simulink model "kalman_filter_design"  (R2023b)
settings: Solver=VariableStepAuto  StartTime=0.0  StopTime=20  MaxStep=0.01  RelTol=1e-3
undefined symbols (not defined in the file): Discrete, Rotation_Local, t_sample, t_sample_camera, Time, Wheel_Speed_to_Motor_Speed
libraries: simulink_extras x5, simulink x4, sharedTrackingLibrary x1, ctrlSharedLib x1
settings Model: Creator=ander  LastModifiedBy=ander

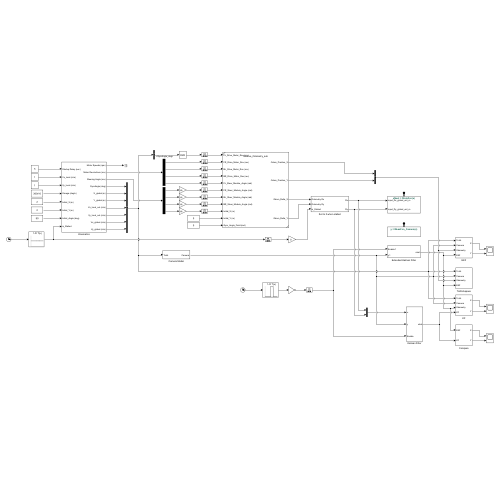
[thumbnail: Simulink's stored preview of the top-level diagram]
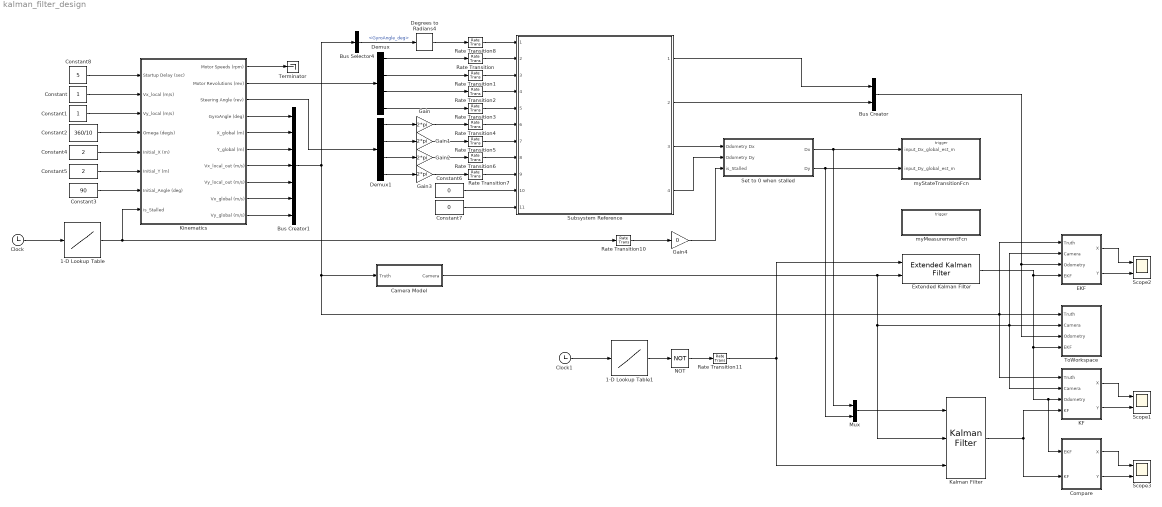
== system kalman_filter_design ==
  1-D Lookup Table : Lookup_n-D  NumberOfTableDimensions=1  BreakpointsForDimension1=[0 7 7.1 10 10.1 15]  Table=[0 0 1 1 0 0]*0  InternalRulePriority=Speed  RndMeth=Simplest
  1-D Lookup Table1 : Lookup_n-D  NumberOfTableDimensions=1  BreakpointsForDimension1=[0 7 7.1 10 10.1 15]  Table=[0 0 1 1 0 0]  InternalRulePriority=Speed  RndMeth=Simplest
  Bus Creator : BusCreator  Inputs=2
  Bus Creator1 : BusCreator  Inputs=7
  Bus Selector4 : BusSelector  OutputSignals=GyroAngle_deg
  Camera Model : Subsystem
  Clock : Clock
  Clock1 : Clock
  Compare : Subsystem
  Constant : Constant
  Constant1 : Constant
  Constant2 : Constant  Value=360/10
  Constant3 : Constant  Value=90
  Constant4 : Constant  Value=2
  Constant5 : Constant  Value=2
  Constant6 : Constant  Value=0
  Constant7 : Constant  Value=0
  Constant8 : Constant  Value=5
  Degrees to Radians4 : simulink_extras/Transformations/Degrees to Radians
  Demux : Demux
  Demux1 : Demux
  EKF : Subsystem
  Extended Kalman Filter : sharedTrackingLibrary/Extended Kalman Filter  StateTransitionFcn=StateFcn  HasStateTransitionJacobianFcn=off  HasAdditiveProcessNoise=Additive  ProcessNoise=1e-3*eye(2)  HasTimeVaryingProcessNoise=off  HasStateTransitionFcnExtraArgument=0  InitialState=[0;0]  InitialStateCovariance=1e-3*eye(2)  MeasurementFcn1=MeasFcn_Camera  HasMeasurementJacobianFcn1=off  HasMeasurementEnablePort1=on  HasAdditiveMeasurementNoise1=Additive  MeasurementNoise1=0.1*eye(2)  HasTimeVaryingMeasurementNoise1=off  HasMeasurementFcnExtraArgument1=0  HasMeasurementWrapping1=off  MeasurementFcn2=MeasFcn_IMU  HasMeasurementJacobianFcn2=off  HasMeasurementEnablePort2=off  HasAdditiveMeasurementNoise2=Additive  MeasurementNoise2=1e-4*eye(2)  HasTimeVaryingMeasurementNoise2=off  HasMeasurementFcnExtraArgument2=0  HasMeasurementWrapping2=off  MeasurementFcn3=myMeasurementFcn  HasMeasurementJacobianFcn3=off  HasMeasurementEnablePort3=off  HasAdditiveMeasurementNoise3=Additive  MeasurementNoise3=1  HasTimeVaryingMeasurementNoise3=off  HasMeasurementFcnExtraArgument3=0  HasMeasurementWrapping3=off  MeasurementFcn4=myMeasurementFcn  HasMeasurementJacobianFcn4=off  HasMeasurementEnablePort4=off  HasAdditiveMeasurementNoise4=Additive  MeasurementNoise4=1  HasTimeVaryingMeasurementNoise4=off  HasMeasurementFcnExtraArgument4=0  HasMeasurementWrapping4=off  MeasurementFcn5=myMeasurementFcn  HasMeasurementJacobianFcn5=off  HasMeasurementEnablePort5=off  HasAdditiveMeasurementNoise5=Additive  MeasurementNoise5=1  HasTimeVaryingMeasurementNoise5=off  HasMeasurementFcnExtraArgument5=0  HasMeasurementWrapping5=off  EnableMultirate=off  StateTransitionFcnSampleTime=t_sample  MeasurementFcn1SampleTime=t_sample_camera  MeasurementFcn2SampleTime=t_sample  MeasurementFcn3SampleTime=1  MeasurementFcn4SampleTime=1  MeasurementFcn5SampleTime=1  UseCurrentEstimator=on  OutputStateCovariance=off  DataType=double  SampleTime=t_sample  NumberOfMeasurements=1
  Gain{,1..3} (4 alike) : Gain  Gain=2*pi
  Gain4 : Gain  Gain=0
  KF : Subsystem
  Kalman Filter : ctrlSharedLib/Kalman Filter  TimeDomain=Discrete-Time  UseCurrentEstimator=on  ModelSource=Individual A, B, C, D matrices  ModelSourceVariable=ss(0.95,1,1,0,1)  A=eye(2)  B=eye(2)  C=eye(2)  D=eye(2)*0  NumberOfStates=1  NumberOfInputs=1  NumberOfOutputs=1  InitialEstimateSource=Dialog  X0=[0;0]  P0=10  UseK=off  UseGH=off  NumberOfProcessNoiseInputs=1  G=eye(2)  TimeInvariantG=on  H=eye(2)*1e-2  TimeInvariantH=on  Q=1e-3*eye(2)  TimeInvariantQ=on  R=0.1*eye(2)  TimeInvariantR=on  N=0  TimeInvariantN=on  AddInputPort=on  AddEnablePort=on  OutputEstimatedY=off  OutputP=off  Ts=-1
  Kinematics : Subsystem
  Mux : Mux  Inputs=2
  NOT : Logic  Operator=NOT  IconShape=distinctive  AllPortsSameDT=off  OutDataTypeStr=boolean
  Rate Transition{,1..8,10..11} (11 alike) : RateTransition  OutPortSampleTime=t_sample
  Scope1 : Scope  NumInputPorts=2
  Scope2 : Scope  NumInputPorts=2
  Scope3 : Scope  NumInputPorts=2
  Set to 0 when stalled : Subsystem
  Subsystem Reference : Subsystem  ReferencedSubsystem=Swerve_Odometry_sub
  Terminator : Terminator
  ToWorkspace : Subsystem
  myMeasurementFcn : Subsystem  TreatAsAtomicUnit=on
  myStateTransitionFcn : Subsystem  TreatAsAtomicUnit=on
  wires:
  Kinematics/2(Motor Revolutions (rev)) -> Demux/1
  Kinematics/1(Motor Speeds (rpm)) -> Terminator/1
  Kinematics/3(Steering Angle (rev)) -> Demux1/1
  Demux/3 -> Rate Transition2/1
  Demux/2 -> Rate Transition1/1
  Demux/4 -> Rate Transition3/1
  Demux/1 -> Rate Transition/1
  Constant3/1 -> Kinematics/7(Initial_Angle (deg))
  Rate Transition/1 -> Subsystem Reference/2
  Rate Transition1/1 -> Subsystem Reference/3
  Rate Transition2/1 -> Subsystem Reference/4
  Rate Transition3/1 -> Subsystem Reference/5
  Rate Transition4/1 -> Subsystem Reference/6
  Rate Transition5/1 -> Subsystem Reference/7
  Rate Transition6/1 -> Subsystem Reference/8
  Rate Transition7/1 -> Subsystem Reference/9
  Rate Transition8/1 -> Subsystem Reference/1
  Constant4/1 -> Kinematics/5(Initial_X (m))
  Constant5/1 -> Kinematics/6(Initial_Y (m))
  Subsystem Reference/1 -> Bus Creator/1
  Bus Creator1/1 -> Bus Selector4/1, KF/1(Truth), EKF/1(Truth), ToWorkspace/1(Truth), Camera Model/1(Truth)
  Bus Creator/1 -> EKF/3(Odometry), ToWorkspace/3(Odometry)
  Demux1/3 -> Gain2/1
  Demux1/2 -> Gain1/1
  Demux1/1 -> Gain/1
  Degrees to Radians4/1 -> Rate Transition8/1
  Gain/1 -> Rate Transition4/1
  Demux1/4 -> Gain3/1
  Gain1/1 -> Rate Transition5/1
  Gain2/1 -> Rate Transition6/1
  Gain3/1 -> Rate Transition7/1
  Extended Kalman Filter/1 -> EKF/4(EKF), KF/3(Odometry), Compare/1(EKF), ToWorkspace/4(EKF)
  EKF/1(X) -> Scope2/1
  EKF/2(Y) -> Scope2/2
  Camera Model/1(Camera) -> Kalman Filter/2, KF/2(Camera), EKF/2(Camera), ToWorkspace/2(Camera), Extended Kalman Filter/2
  Constant6/1 -> Subsystem Reference/10
  Constant7/1 -> Subsystem Reference/11
  Bus Selector4/1 -> Degrees to Radians4/1  "<GyroAngle_deg>"
  Clock/1 -> 1-D Lookup Table/1
  Kinematics/8(Vy_local_out (m/s)) -> Bus Creator1/5
  Kinematics/7(Vx_local_out (m/s)) -> Bus Creator1/4
  Kinematics/9(Vx_global (m/s)) -> Bus Creator1/6
  Kinematics/10(Vy_global (m/s)) -> Bus Creator1/7
  Kinematics/4(GyroAngle (deg)) -> Bus Creator1/1
  Kinematics/5(X_global (m)) -> Bus Creator1/2
  Kinematics/6(Y_global (m)) -> Bus Creator1/3
  Constant2/1 -> Kinematics/4(Omega (deg/s))
  Constant/1 -> Kinematics/2(Vx_local (m/s))
  Constant1/1 -> Kinematics/3(Vy_local (m/s))
  Constant8/1 -> Kinematics/1(Startup Delay (sec))
  1-D Lookup Table/1 -> Kinematics/8(is_Stalled), Rate Transition10/1
  Mux/1 -> Kalman Filter/1
  Kalman Filter/1 -> KF/4(KF), Compare/2(KF)
  KF/2(Y) -> Scope1/2
  KF/1(X) -> Scope1/1
  Set to 0 when stalled/1(Dx) -> Mux/1, myStateTransitionFcn/1(input_Dx_global_est_m)
  Set to 0 when stalled/2(Dy) -> Mux/2, myStateTransitionFcn/2(input_Dy_global_est_m)
  Rate Transition10/1 -> Gain4/1
  Gain4/1 -> Set to 0 when stalled/3(is_Stalled)
  Subsystem Reference/2 -> Bus Creator/2
  Subsystem Reference/3 -> Set to 0 when stalled/1(Odometry Dx)
  Subsystem Reference/4 -> Set to 0 when stalled/2(Odometry Dy)
  Clock1/1 -> 1-D Lookup Table1/1
  1-D Lookup Table1/1 -> NOT/1
  NOT/1 -> Rate Transition11/1
  Rate Transition11/1 -> Kalman Filter/3, Extended Kalman Filter/1
  Compare/1(X) -> Scope3/1
  Compare/2(Y) -> Scope3/2

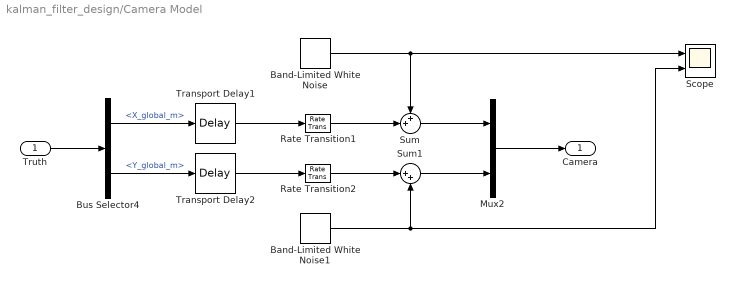
== system kalman_filter_design/Camera Model ==
  Truth : Inport
  Band-Limited White Noise : simulink/Sources/Band-Limited White Noise  Cov=1e-4  Ts=t_sample_camera  seed=[23341]
  Band-Limited White Noise1 : simulink/Sources/Band-Limited White Noise  Cov=1e-4  Ts=t_sample_camera  seed=[23342]
  Bus Selector4 : BusSelector  OutputSignals=X_global_m,Y_global_m
  Mux2 : Mux  Inputs=2
  Rate Transition1 : RateTransition  OutPortSampleTime=t_sample
  Rate Transition2 : RateTransition  OutPortSampleTime=t_sample
  Scope : Scope  NumInputPorts=2
  Sum : Sum  Inputs=++|
  Sum1 : Sum  Inputs=|++
  Transport Delay1 : TransportDelay  DelayTime=0.1
  Transport Delay2 : TransportDelay  DelayTime=0.1
  Camera : Outport
  wires:
  Mux2/1 -> Camera/1
  Truth/1 -> Bus Selector4/1
  Bus Selector4/1 -> Transport Delay1/1  "<X_global_m>"
  Bus Selector4/2 -> Transport Delay2/1  "<Y_global_m>"
  Transport Delay1/1 -> Rate Transition1/1
  Transport Delay2/1 -> Rate Transition2/1
  Rate Transition1/1 -> Sum/2
  Band-Limited White Noise/1 -> Scope/1, Sum/1
  Rate Transition2/1 -> Sum1/1
  Band-Limited White Noise1/1 -> Scope/2, Sum1/2
  Sum/1 -> Mux2/1
  Sum1/1 -> Mux2/2

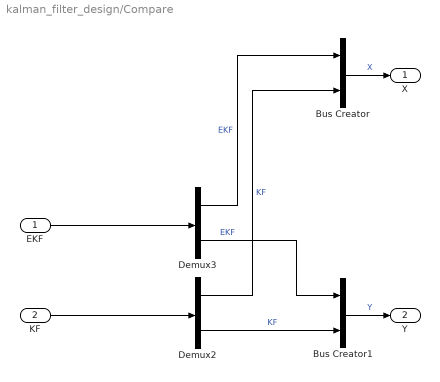
== system kalman_filter_design/Compare ==
  EKF : Inport
  KF : Inport  Port=2
  Bus Creator : BusCreator  Inputs=2
  Bus Creator1 : BusCreator  Inputs=2
  Demux2 : Demux  Outputs=2
  Demux3 : Demux  Outputs=2
  X : Outport
  Y : Outport  Port=2
  wires:
  Demux2/2 -> Bus Creator1/2  "KF"
  Bus Creator/1 -> X/1  "X"
  Demux2/1 -> Bus Creator/2  "KF"
  Bus Creator1/1 -> Y/1  "Y"
  KF/1 -> Demux2/1
  EKF/1 -> Demux3/1
  Demux3/1 -> Bus Creator/1  "EKF"
  Demux3/2 -> Bus Creator1/1  "EKF"

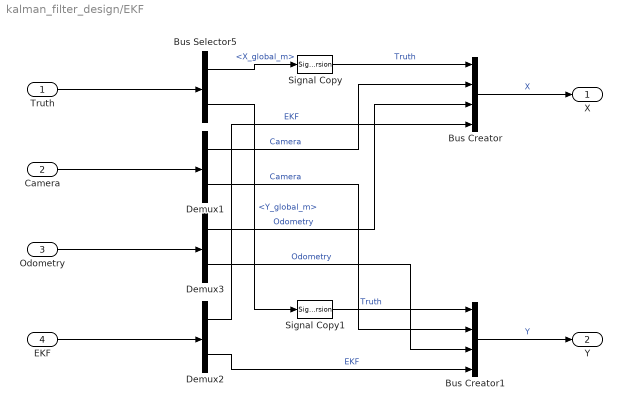
== system kalman_filter_design/EKF ==
  Truth : Inport
  Camera : Inport  Port=2
  Odometry : Inport  Port=3
  EKF : Inport  Port=4
  Bus Creator : BusCreator  Inputs=4
  Bus Creator1 : BusCreator  Inputs=4
  Bus Selector5 : BusSelector  OutputSignals=X_global_m,Y_global_m
  Demux1 : Demux  Outputs=2
  Demux2 : Demux  Outputs=2
  Demux3 : Demux  Outputs=2
  Signal Copy : SignalConversion  OverrideOpt=off
  Signal Copy1 : SignalConversion  OverrideOpt=off
  X : Outport
  Y : Outport  Port=2
  wires:
  Signal Copy1/1 -> Bus Creator1/1  "Truth"
  Signal Copy/1 -> Bus Creator/1  "Truth"
  Truth/1 -> Bus Selector5/1
  Demux2/2 -> Bus Creator1/4  "EKF"
  Bus Selector5/1 -> Signal Copy/1  "<X_global_m>"
  Bus Creator/1 -> X/1  "X"
  Demux2/1 -> Bus Creator/4  "EKF"
  Bus Selector5/2 -> Signal Copy1/1  "<Y_global_m>"
  Bus Creator1/1 -> Y/1  "Y"
  Camera/1 -> Demux1/1
  Demux1/1 -> Bus Creator/2  "Camera"
  Demux1/2 -> Bus Creator1/2  "Camera"
  EKF/1 -> Demux2/1
  Odometry/1 -> Demux3/1
  Demux3/1 -> Bus Creator/3  "Odometry"
  Demux3/2 -> Bus Creator1/3  "Odometry"

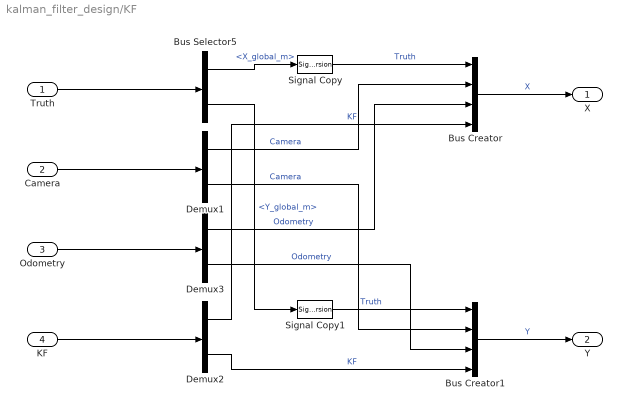
== system kalman_filter_design/KF ==
  Truth : Inport
  Camera : Inport  Port=2
  Odometry : Inport  Port=3
  KF : Inport  Port=4
  Bus Creator : BusCreator  Inputs=4
  Bus Creator1 : BusCreator  Inputs=4
  Bus Selector5 : BusSelector  OutputSignals=X_global_m,Y_global_m
  Demux1 : Demux  Outputs=2
  Demux2 : Demux  Outputs=2
  Demux3 : Demux  Outputs=2
  Signal Copy : SignalConversion  OverrideOpt=off
  Signal Copy1 : SignalConversion  OverrideOpt=off
  X : Outport
  Y : Outport  Port=2
  wires:
  Demux3/2 -> Bus Creator1/3  "Odometry"
  Demux3/1 -> Bus Creator/3  "Odometry"
  Odometry/1 -> Demux3/1
  KF/1 -> Demux2/1
  Demux1/2 -> Bus Creator1/2  "Camera"
  Demux1/1 -> Bus Creator/2  "Camera"
  Camera/1 -> Demux1/1
  Bus Creator1/1 -> Y/1  "Y"
  Bus Selector5/2 -> Signal Copy1/1  "<Y_global_m>"
  Demux2/1 -> Bus Creator/4  "KF"
  Bus Creator/1 -> X/1  "X"
  Bus Selector5/1 -> Signal Copy/1  "<X_global_m>"
  Demux2/2 -> Bus Creator1/4  "KF"
  Truth/1 -> Bus Selector5/1
  Signal Copy/1 -> Bus Creator/1  "Truth"
  Signal Copy1/1 -> Bus Creator1/1  "Truth"

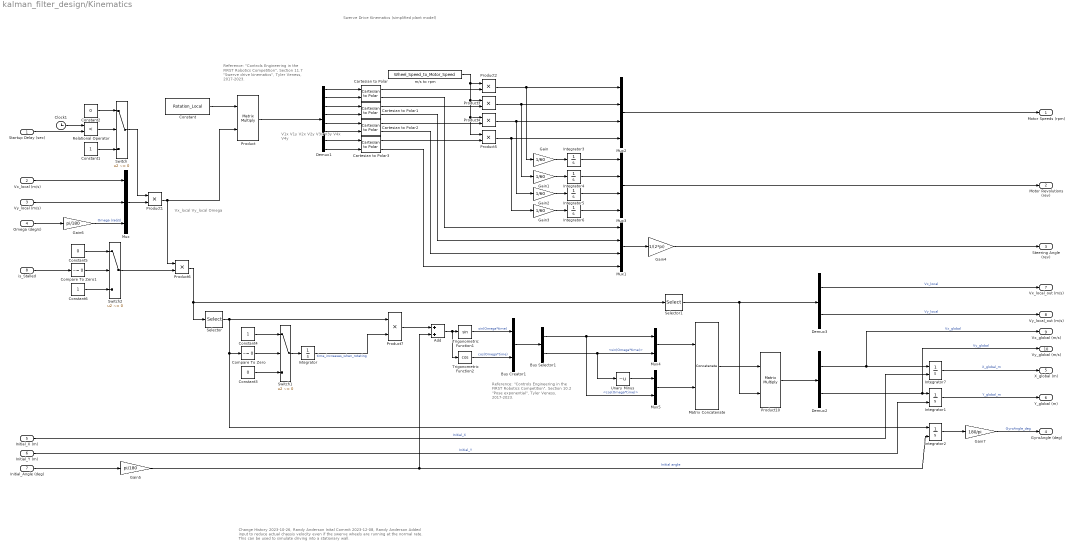
== system kalman_filter_design/Kinematics ==
  note: Swerve Drive Kinematics
      | (simplified plant model)
  note: Vx_local
      | Vy_local
      | Omega
  note: V1x
      | V1y
      | V2x
      | V2y
      | V3x
      | V3y
      | V4x
      | V4y
  note: Reference: "Controls Engineering in the
      |  FIRST Robotics Competition",
      | Section 11.7 "Swerve drive kinematics",
      | Tyler Veness, 2017-2023.
  note: Reference: "Controls Engineering in the
      |  FIRST Robotics Competition",
      | Section 10.2 "Pose exponential",
      | Tyler Veness, 2017-2023.
  note: Change History
      | 2023-10-26, Randy Anderson
      | Inital Commit
      | 2023-12-08, Randy Anderson
      | Added input to reduce actual chassis velocity even if the swerve wheels are running at
      | the normal rate. This can be used to simulate driving into a stationary wall.
  Startup Delay (sec) : Inport
  Vx_local (m/s) : Inport  Port=2
  Vy_local (m/s) : Inport  Port=3
  Omega (deg/s) : Inport  Port=4
  Initial_X (m) : Inport  Port=5
  Initial_Y (m) : Inport  Port=6
  Initial_Angle (deg) : Inport  Port=7
  is_Stalled : Inport  Port=8
  Add : Sum
  Bus Creator1 : BusCreator  Inputs=2
  Bus Selector1 : BusSelector  OutputSignals=cos(Omega*time),sin(Omega*time)
  Cartesian to Polar{,1..3} (4 alike) : simulink_extras/Transformations/Cartesian to Polar
  Clock1 : Clock
  Compare To Zero : simulink/Logic and Bit Operations/Compare To Zero  relop=~=  OutDataTypeStr=boolean
  Compare To Zero1 : simulink/Logic and Bit Operations/Compare To Zero  relop=~=  OutDataTypeStr=boolean
  Constant : Constant  Value=Rotation_Local
  Constant1 : Constant
  Constant2 : Constant  Value=0
  Constant3 : Constant  Value=0
  Constant4 : Constant
  Constant5 : Constant  Value=0
  Constant6 : Constant
  Demux1 : Demux  Outputs=8
  Demux2 : Demux  Outputs=2
  Demux3 : Demux  Outputs=2
  Gain{,1..3} (4 alike) : Gain  Gain=1/60
  Gain4 : Gain  Gain=1/(2*pi)
  Gain5 : Gain  Gain=pi/180
  Gain6 : Gain  Gain=pi/180
  Gain7 : Gain  Gain=180/pi
  Integrator{,3..6} (5 alike) : Integrator
  Integrator1 : Integrator  InitialConditionSource=external
  Integrator2 : Integrator  InitialConditionSource=external
  Integrator7 : Integrator  InitialConditionSource=external
  Matrix Concatenate : Concatenate  Mode=Multidimensional array  ConcatenateDimension=2
  Mux : Mux  Inputs=3
  Mux1 : Mux
  Mux2 : Mux
  Mux3 : Mux
  Mux4 : Mux  Inputs=2
  Mux5 : Mux  Inputs=2
  Product : Product  Multiplication=Matrix(*)
  Product{1..7} (7 alike) : Product
  Product10 : Product  Multiplication=Matrix(*)
  Relational Operator : RelationalOperator  Operator=<  OutDataTypeStr=boolean  RndMeth=Simplest  InputSameDT=off
  Selector : Selector  InputPortWidth=3  IndexOptions=Index vector (dialog)  Indices=3  OutputSizes=1
  Selector1 : Selector  InputPortWidth=3  IndexOptions=Index vector (dialog)  Indices=[1 2]  OutputSizes=1
  Switch : Switch  Criteria=u2 ~= 0  SaturateOnIntegerOverflow=off  InputSameDT=off
  Switch1 : Switch  Criteria=u2 ~= 0  SaturateOnIntegerOverflow=off  InputSameDT=off
  Switch2 : Switch  Criteria=u2 ~= 0  SaturateOnIntegerOverflow=off  InputSameDT=off
  Trigonometric Function1 : Trigonometry
  Trigonometric Function2 : Trigonometry  Operator=cos
  Unary Minus : UnaryMinus
  m/s to rpm : Constant  Value=Wheel_Speed_to_Motor_Speed
  Motor Speeds (rpm) : Outport
  Motor Revolutions (rev) : Outport  Port=2
  Steering Angle (rev) : Outport  Port=3
  GyroAngle (deg) : Outport  Port=4
  X_global (m) : Outport  Port=5
  Y_global (m) : Outport  Port=6
  Vx_local_out (m/s) : Outport  Port=7
  Vy_local_out (m/s) : Outport  Port=8
  Vx_global (m/s) : Outport  Port=9
  Vy_global (m/s) : Outport  Port=10
  wires:
  Demux1/2 -> Cartesian to Polar/2
  Integrator6/1 -> Mux3/4
  Integrator5/1 -> Mux3/3
  Product/1 -> Demux1/1
  Cartesian to Polar1/2 -> Mux1/2
  m/s to rpm/1 -> Product5/1, Product4/1, Product3/1, Product2/1
  Constant/1 -> Product/1
  Demux1/8 -> Cartesian to Polar3/2
  Demux1/7 -> Cartesian to Polar3/1
  Demux1/3 -> Cartesian to Polar1/1
  Cartesian to Polar1/1 -> Product3/2
  Product1/1 -> Product/2, Product6/1
  Mux2/1 -> Motor Speeds (rpm)/1
  Integrator4/1 -> Mux3/2
  Vy_local (m/s)/1 -> Mux/2
  Mux3/1 -> Motor Revolutions (rev)/1
  Gain/1 -> Integrator3/1
  Demux1/1 -> Cartesian to Polar/1
  Cartesian to Polar3/2 -> Mux1/4
  Demux1/5 -> Cartesian to Polar2/1
  Omega (deg/s)/1 -> Gain6/1
  Product3/1 -> Gain1/1, Mux2/2
  Cartesian to Polar2/2 -> Mux1/3
  Cartesian to Polar2/1 -> Product4/2
  Product5/1 -> Gain3/1, Mux2/4
  Integrator3/1 -> Mux3/1
  Demux1/4 -> Cartesian to Polar1/2
  Cartesian to Polar/1 -> Product2/2
  Mux1/1 -> Gain4/1
  Vx_local (m/s)/1 -> Mux/1
  Gain2/1 -> Integrator5/1
  Cartesian to Polar/2 -> Mux1/1
  Gain4/1 -> Steering Angle (rev)/1
  Product4/1 -> Gain2/1, Mux2/3
  Product2/1 -> Gain/1, Mux2/1
  Demux1/6 -> Cartesian to Polar2/2
  Cartesian to Polar3/1 -> Product5/2
  Gain1/1 -> Integrator4/1
  Gain3/1 -> Integrator6/1
  Mux4/1 -> Matrix Concatenate/1
  Trigonometric Function1/1 -> Bus Creator1/1  "sin(Omega*time)"
  Trigonometric Function2/1 -> Bus Creator1/2  "cos(Omega*time)"
  Bus Creator1/1 -> Bus Selector1/1
  Mux5/1 -> Matrix Concatenate/2
  Matrix Concatenate/1 -> Product10/1
  Product10/1 -> Demux2/1
  Bus Selector1/1 -> Mux4/1, Mux5/2  "<cos(Omega*time)>"
  Bus Selector1/2 -> Mux4/2, Unary Minus/1  "<sin(Omega*time)>"
  Unary Minus/1 -> Mux5/1
  Integrator7/1 -> X_global (m)/1  "X_global_m"
  Integrator1/1 -> Y_global (m)/1  "Y_global_m"
  Integrator2/1 -> Gain7/1
  Gain6/1 -> Mux/3  "Omega (rad/s)"
  Add/1 -> Trigonometric Function2/1, Trigonometric Function1/1
  Product7/1 -> Add/1
  Initial_Angle (deg)/1 -> Gain5/1
  Initial_X (m)/1 -> Integrator7/2  "Initial_X"
  Initial_Y (m)/1 -> Integrator1/2  "Initial_Y"
  Demux2/1 -> Vx_global (m/s)/1, Integrator7/1  "Vx_global"
  Demux2/2 -> Vy_global (m/s)/1, Integrator1/1  "Vy_global"
  Selector1/1 -> Product10/2, Demux3/1
  Product6/1 -> Selector1/1, Selector/1
  Demux3/1 -> Vx_local_out (m/s)/1  "Vx_local"
  Demux3/2 -> Vy_local_out (m/s)/1  "Vy_local"
  Clock1/1 -> Relational Operator/1
  Startup Delay (sec)/1 -> Relational Operator/2
  Relational Operator/1 -> Switch/2
  Constant1/1 -> Switch/3
  Constant2/1 -> Switch/1
  Mux/1 -> Product1/2
  Switch/1 -> Product1/1
  Selector/1 -> Integrator2/1, Compare To Zero/1, Product7/1
  Gain7/1 -> GyroAngle (deg)/1  "GyroAngle_deg"
  Gain5/1 -> Add/2, Integrator2/2  "Initial angle"
  Compare To Zero/1 -> Switch1/2
  Constant3/1 -> Switch1/3
  Constant4/1 -> Switch1/1
  Switch1/1 -> Integrator/1
  Integrator/1 -> Product7/2  "time_increases_when_rotating"
  Compare To Zero1/1 -> Switch2/2
  is_Stalled/1 -> Compare To Zero1/1
  Switch2/1 -> Product6/2
  Constant5/1 -> Switch2/1
  Constant6/1 -> Switch2/3

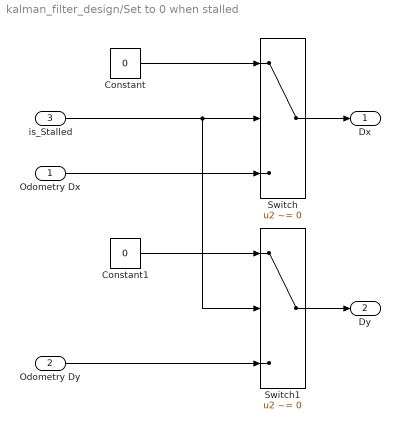
== system kalman_filter_design/Set to 0 when stalled ==
  Odometry Dx : Inport
  Odometry Dy : Inport  Port=2
  is_Stalled : Inport  Port=3
  Constant : Constant  Value=0
  Constant1 : Constant  Value=0
  Switch : Switch  Criteria=u2 ~= 0  SaturateOnIntegerOverflow=off  InputSameDT=off
  Switch1 : Switch  Criteria=u2 ~= 0  SaturateOnIntegerOverflow=off  InputSameDT=off
  Dx : Outport
  Dy : Outport  Port=2
  wires:
  Odometry Dx/1 -> Switch/3
  Switch/1 -> Dx/1
  Switch1/1 -> Dy/1
  Odometry Dy/1 -> Switch1/3
  Constant/1 -> Switch/1
  Constant1/1 -> Switch1/1
  is_Stalled/1 -> Switch1/2, Switch/2

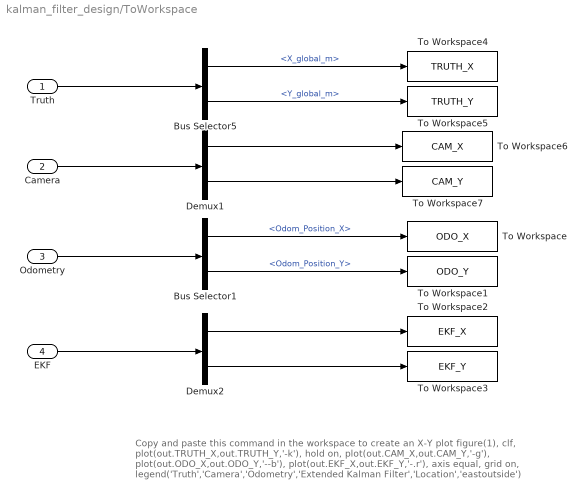
== system kalman_filter_design/ToWorkspace ==
  note: Copy and paste this command in the workspace to create an X-Y plot
      |
      | figure(1), clf, plot(out.TRUTH_X,out.TRUTH_Y,'-k'), hold on, plot(out.CAM_X,out.CAM_Y,'-g'), plot(out.ODO_X,out.ODO_Y,'--b'), plot(out.EKF_X,out.EKF_Y,'-.r'), axis equal, grid on, legend('Truth','Camera','Odometry','Extended Kalman Filter','Location','eastoutside')
  Truth : Inport
  Camera : Inport  Port=2
  Odometry : Inport  Port=3
  EKF : Inport  Port=4
  Bus Selector1 : BusSelector  OutputSignals=Odom_Position_X,Odom_Position_Y
  Bus Selector5 : BusSelector  OutputSignals=X_global_m,Y_global_m
  Demux1 : Demux  Outputs=2
  Demux2 : Demux  Outputs=2
  To Workspace : ToWorkspace  VariableName=ODO_X  SampleTime=-1
  To Workspace1 : ToWorkspace  VariableName=ODO_Y  SampleTime=-1
  To Workspace2 : ToWorkspace  VariableName=EKF_X  SampleTime=-1
  To Workspace3 : ToWorkspace  VariableName=EKF_Y  SampleTime=-1
  To Workspace4 : ToWorkspace  VariableName=TRUTH_X  SampleTime=-1
  To Workspace5 : ToWorkspace  VariableName=TRUTH_Y  SampleTime=-1
  To Workspace6 : ToWorkspace  VariableName=CAM_X  SampleTime=-1
  To Workspace7 : ToWorkspace  VariableName=CAM_Y  SampleTime=-1
  wires:
  EKF/1 -> Demux2/1
  Camera/1 -> Demux1/1
  Truth/1 -> Bus Selector5/1
  Odometry/1 -> Bus Selector1/1
  Bus Selector1/1 -> To Workspace/1  "<Odom_Position_X>"
  Bus Selector1/2 -> To Workspace1/1  "<Odom_Position_Y>"
  Demux2/1 -> To Workspace2/1
  Demux2/2 -> To Workspace3/1
  Bus Selector5/1 -> To Workspace4/1  "<X_global_m>"
  Bus Selector5/2 -> To Workspace5/1  "<Y_global_m>"
  Demux1/1 -> To Workspace6/1
  Demux1/2 -> To Workspace7/1

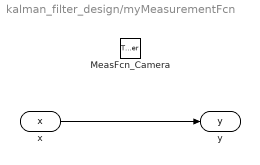
== system kalman_filter_design/myMeasurementFcn ==
  MeasFcn_Camera : TriggerPort  TriggerType=function-call  IsSimulinkFunction=on  FunctionName=MeasFcn_Camera  FunctionVisibility=scoped  VariantControl=(inherit)
  x : ArgIn  DisableCoverage=on  PortDimensions=2  ArgumentName=x
  y : ArgOut  DisableCoverage=on  PortDimensions=2  ArgumentName=y
  wires:
  x/1 -> y/1

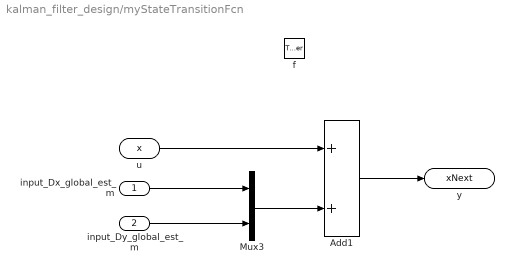
== system kalman_filter_design/myStateTransitionFcn ==
  input_Dx_global_est_m : Inport
  input_Dy_global_est_m : Inport  Port=2
  f : TriggerPort  TriggerType=function-call  IsSimulinkFunction=on  FunctionName=StateFcn  FunctionVisibility=scoped  VariantControl=(inherit)
  Add1 : Sum
  Mux3 : Mux  Inputs=2
  u : ArgIn  DisableCoverage=on  PortDimensions=2  ArgumentName=x
  y : ArgOut  DisableCoverage=on  PortDimensions=2  ArgumentName=xNext
  wires:
  input_Dx_global_est_m/1 -> Mux3/1
  input_Dy_global_est_m/1 -> Mux3/2
  Add1/1 -> y/1
  Mux3/1 -> Add1/2
  u/1 -> Add1/1
